simulink model "Golf_Lin_Classique"  (R2019a)
settings: Solver=VariableStepAuto  StartTime=0.0  StopTime=700  RelTol=1e-3
values from neighbouring files (symbols this model uses):
  DEG2RAD = pi/180.    (= 0.0174532925199)    [mainProjetCADV_2a.m]    (also in utAcDynamicsFunction.m; utConstantAeroCoeff.m)
  RAD2DEG = 180/pi    (= 57.2957795131)    [mainProjetCADV_2a.m]    (also in utAcDynamicsFunction.m)
  thetaTrim = trimVal(3)    [mainProjetCADV_2a.m]
undefined symbols (not defined in the file or in its folder): Cpf, Kd, Ki, Kp, state4den, state4num
libraries: simulink x1
settings Model: Creator=bourdiul  LastModifiedBy=mariu

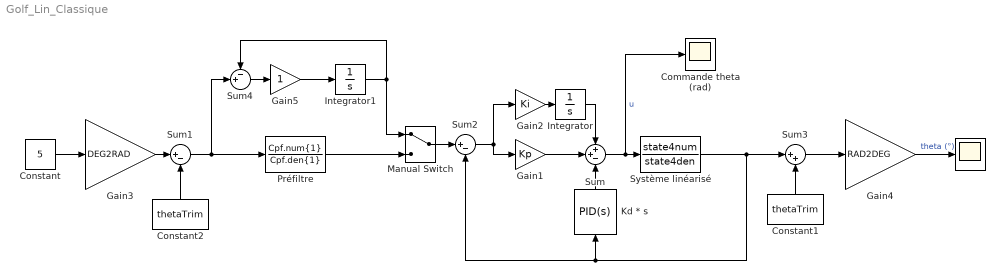
== system Golf_Lin_Classique ==
  " " : Scope
  Commande theta (rad) : Scope
  Constant : Constant  Value=5
  Constant1 : Constant  Value=thetaTrim
  Constant2 : Constant  Value=thetaTrim
  Gain1 : Gain  Gain=Kp
  Gain2 : Gain  Gain=Ki
  Gain3 : Gain  Gain=DEG2RAD
  Gain4 : Gain  Gain=RAD2DEG
  Gain5 : Gain
  Integrator : Integrator
  Integrator1 : Integrator
  Kd * s : simulink/Continuous/PID Controller  Controller=PID  Form=Parallel  TimeDomain=Continuous-time  SampleTime=-1  IntegratorMethod=Forward Euler  FilterMethod=Forward Euler  ControllerParametersSource=internal  P=0  I=0  D=Kd  UseFilter=on  N=100  TunerSelectOption=Transfer Function Based (PID Tuner App)  InitialConditionSource=internal  InitialConditionForIntegrator=0  InitialConditionForFilter=0  DifferentiatorICPrevScaledInput=0  ExternalReset=none  TrackingMode=off  Kt=1  LimitOutput=off  UpperSaturationLimit=inf  LowerSaturationLimit=-inf  LinearizeAsGain=on  AntiWindupMode=none  Kb=1  POutMin=[]  POutMax=[]  IOutMin=[]  IOutMax=[]  DOutMin=[]  DOutMax=[]  NOutMin=[]  NOutMax=[]  SumOutMin=[]  SumOutMax=[]  SaturationOutMin=[]  SaturationOutMax=[]  PParamMin=[]  PParamMax=[]  IParamMin=[]  IParamMax=[]  DParamMin=[]  DParamMax=[]  NParamMin=[]  NParamMax=[]  KbParamMin=[]  KbParamMax=[]  KtParamMin=[]  KtParamMax=[]  KbOutMin=[]  KbOutMax=[]  KtOutMin=[]  KtOutMax=[]  IntegratorOutMin=[]  IntegratorOutMax=[]  FilterOutMin=[]  FilterOutMax=[]  SumI1OutMin=[]  SumI1OutMax=[]  SumI2OutMin=[]  SumI2OutMax=[]  SumI3OutMin=[]  SumI3OutMax=[]  SumI4OutMin=[]  SumI4OutMax=[]  SumDOutMin=[]  SumDOutMax=[]  DifferentiatorOutMin=[]  DifferentiatorOutMax=[]  FilterDiffOutCoefMin=[]  FilterDiffOutCoefMax=[]  ReciprocalOutMin=[]  ReciprocalOutMax=[]  SumDenOutMin=[]  SumDenOutMax=[]  SumNumOutMin=[]  SumNumOutMax=[]  DivideOutMin=[]  DivideOutMax=[]  IntegratorContinuousStateAttributes=''  IntegratorStateMustResolveToSignalObject=off  IntegratorRTWStateStorageClass=Auto  FilterContinuousStateAttributes=''  FilterStateMustResolveToSignalObject=off  FilterRTWStateStorageClass=Auto  ParallelPVariant=InternalParameters  IdealPVariant=Disabled  IVariant=InternalParameters  DVariant=InternalParameters  IntegratorVariant=Continuous  SatVariant=Disabled  AWVariant=Passthrough  PCopyVariant=Disabled  TRVariant=Disabled  FdbkBlocksVariant=Forward  IdealPFdbkVariant=Disabled  SatFdbkVariant=Disabled  DerivativeFilterVariant=ContFilter  NVariant=InternalParameters  NCopyVariant=Disabled  FilterICVariant=InternalICsFilter  IntegratorICVariant=InternalICs  ExternalResetVariant=Disabled  TRSumVariant=Passthrough  SumFdbkVariant=Disabled  SumVariant=Sum_PID
  Manual Switch : ManualSwitch
  Préfiltre : TransferFcn  Numerator=Cpf.num{1}  Denominator=Cpf.den{1}
  Sum : Sum  Inputs=++-
  Sum1 : Sum  Inputs=|+-
  Sum2 : Sum  Inputs=|+-
  Sum3 : Sum  Inputs=|++
  Sum4 : Sum  Inputs=-+|
  Système linéarisé : TransferFcn  Numerator=state4num  Denominator=state4den
  wires:
  Système linéarisé/1 -> Sum2/2, Kd * s/1, Sum3/1
  Sum/1 -> Commande theta (rad)/1, Système linéarisé/1  "u"
  Kd * s/1 -> Sum/3
  Sum1/1 -> Sum4/2, Préfiltre/1
  Sum2/1 -> Gain1/1, Gain2/1
  Gain1/1 -> Sum/2
  Gain2/1 -> Integrator/1
  Integrator/1 -> Sum/1
  Constant1/1 -> Sum3/2
  Constant2/1 -> Sum1/2
  Gain3/1 -> Sum1/1
  Sum3/1 -> Gain4/1
  Gain4/1 -> " "/1  "theta (°)"
  Sum4/1 -> Gain5/1
  Gain5/1 -> Integrator1/1
  Préfiltre/1 -> Manual Switch/2
  Manual Switch/1 -> Sum2/1
  Integrator1/1 -> Manual Switch/1, Sum4/1
  Constant/1 -> Gain3/1
